simulink model "mltvlib_tvgain"  (R2018b)
settings: Solver=VariableStepAuto  StartTime=0.0  StopTime=10.0  RelTol=1e-3
undefined symbols (not defined in the file or in its folder): K
libraries: ltvlib x2
settings Model: Creator=jyotbuch  LastModifiedBy=jyotbuch

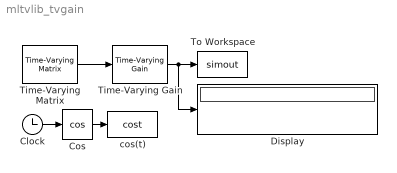
== system mltvlib_tvgain ==
  Clock : Clock
  Cos : Trigonometry  Operator=cos
  Display : Display
  Time-Varying Gain : ltvlib/Time-Varying Gain  K=K
      settings: SourceProductName=Linear Time-Varying Systems Toolbox
  Time-Varying Matrix : ltvlib/Time-Varying Matrix  M=inMAT  vec1D=on
      settings: SourceProductName=Linear Time-Varying Systems Toolbox
  To Workspace : ToWorkspace  VariableName=simout  SampleTime=-1
  cos(t) : ToWorkspace  VariableName=cost  SampleTime=-1
  wires:
  Time-Varying Matrix/1 -> Time-Varying Gain/1
  Clock/1 -> Cos/1
  Cos/1 -> cos(t)/1
  Time-Varying Gain/1 -> Display/1, To Workspace/1
